simulink model "feed_system_harness_fuel_25a"  (R2025a)
settings: Solver=VariableStepAuto  StartTime=0  StopTime=10  RelTol=1e-3
values from neighbouring files (symbols this model uses):
  Kp1 = min(Kp2, 10)    [tuningAlgorithm.m]
  Kp2 = Kp    [tuningAlgorithm.m]
  P_prop_ethanol = [1 2 3 4 5 6 7 8 9 10 11 12 ... (100 elements, 1x100)]    [simscape_fluids_data.mat]
  T_prop_ethanol = [0 2 4 6 8 10 12 14 16 18 20 22 ... (51 elements, 1x51)]    [simscape_fluids_data.mat]
  T_prop_n2 = [-100 -99 -98 -97 -96 -95 -94 -93 -92 -91 -90 -89 ... (201 elements, 1x201)]    [simscape_fluids_data.mat]
libraries: fl_lib x31, nesl_utility x20, simulink x5, SimscapeFluids_lib x4, slpidlib x1
(part 2 of 2)

== matlab function feed_system_harness_fuel_25a/FeedBack Command ==
  data: propPressure input; valveAngle output; nd_error output; Kp input
function [valveAngle, nd_error] = eregControl(propPressure, Kp)

pressureSetpoint = 60e+05;
nd_error = (1 - propPressure/pressureSetpoint); %Non dimensional error
theta = nd_error * Kp;  %In degrees

valveAngle = deg2rad(theta);

== matlab function feed_system_harness_fuel_25a/FeedForwardCommand ==
  data: n2Pressure input; valveAngle output; CdA output; CdACorrectionFactor input; CdAArray input
function [valveAngle, CdA] = feedForwardAngle(n2Pressure, CdACorrectionFactor, CdAArray)

    mdotProp = 0.7645;
    rhoProp = 786;
    % Required effective flow area
    CdA = (mdotProp / rhoProp) * 1/sqrt(max(0,n2Pressure)) * 0.673;
% Ball valve opening angle [deg]
    thetaArray = [0, 10, 20, 30, 40, 50, 60, 70, 80, 90];
% Approximate effective CdA for 6 mm bore ball valve [m^2]
    CdAArray = CdAArray*CdACorrectionFactor;
    theta = 0;

    % Clamp
    if CdA <= CdAArray(1)

        theta = thetaArray(1);

    elseif CdA >= CdAArray(end)

        theta = thetaArray(end);

    else

        % Linear interpolation between LUT points
        for i = 1:length(CdAArray)-1

            if CdA >= CdAArray(i) && CdA <= CdAArray(i+1)

                theta = thetaArray(i) + ...
                    ((CdA - CdAArray(i)) / ...
                    (CdAArray(i+1) - CdAArray(i))) * ...
                    (thetaArray(i+1) - thetaArray(i));

                break;

            end

        end

    end

    % Output angle in radians
    valveAngle = deg2rad(theta);

end

== matlab function feed_system_harness_fuel_25a/CdA Robustness Function ==
  data: array output; shiftBool input; shiftIdx input; scaleFactor input
function array = CdAArray(shiftBool, shiftIdx, scaleFactor)
array   = [0, 0, 0, 4.0e-6, 12.7e-6, 15.2e-6, 17.1e-6, 18.6e-6, 19.5e-6, 19.8e-6];
array = array * scaleFactor;
if shiftBool == true
    array = shiftArray(array, shiftIdx);
end

end

function shifted = shiftArray(array, n)
    % Shifts array by n positions.
    %   n > 0: shifts forward (right), padding the start with the first value
    %   n < 0: shifts backward (left), padding the end with the last value
    %   n = 0: returns array unchanged

    N = numel(array);
    shifted = zeros(size(array));

    if n >= 0
        n = min(n, N);
        shifted(1:n) = array(1);                  % pad start with first value
        shifted(n+1:end) = array(1:N-n);
    else
        n = min(-n, N);
        shifted(1:N-n) = array(n+1:end);
        shifted(N-n+1:end) = array(end);           % pad end with last value
    end
end
